simulink model "AppMain"  (R2021a)
settings: Solver=FixedStepDiscrete  StartTime=0.0  StopTime=0.02  FixedStep=10e-3  RelTol=1e-3
PreLoadFcn:
  | AppMain_data
values from neighbouring files (symbols this model uses):
  CtrlConst = struct    [AppMain_data.m]
  TaskTimeBase = struct    [AppMain_data.m]
undefined symbols (not defined in the file or in its folder): Lock, Open, Short
libraries: simulink x18, lib1 x6
(part 1 of 2)
settings Model: Creator=mdl4347  LastModifiedBy=13714
settings SolverCC: AlgebraicLoopSolver=TrustRegion
settings DataIOCC: ReturnWorkspaceOutputs=off
settings OptimizationCC: DefaultParameterBehavior=Inlined  InlineInvariantSignals=on  BufferReuse=off  GlobalBufferReuse=off  PassReuseOutputArgsAs=Individual arguments  OptimizeBlockOrder=speed  DifferentSizesBufferReuse=on  LabelGuidedReuse=on  EfficientTunableParamExpr=on
settings DebuggingCC: WriteAfterWriteMsg=EnableAllAsError  AlgebraicLoopMsg=error  IntegerOverflowMsg=error  ParameterUnderflowMsg=error  ParameterTunabilityLossMsg=error  BusObjectLabelMismatch=error  AllowSymbolicDim=off  ModelReferenceIOMsg=warning  PregeneratedLibrarySubsystemCodeDiagnostic=none  StrictBusMsg=ErrorOnBusTreatedAsVector  NonBusSignalsTreatedAsBus=error  SFInvalidInputDataAccessInChartInitDiag=error  SFTransitionOutsideNaturalParentDiag=error  SFUnreachableExecutionPathDiag=error  SFUndirectedBroadcastEventsDiag=error  SFTransitionActionBeforeConditionDiag=error  SFMachineParentedDataDiag=warning  IntegerSaturationMsg=error  ArithmeticOperatorsInVariantConditions=warning
settings HardwareCC: ProdBitPerPointer=32  ProdBitPerSizeT=32  ProdBitPerPtrDiffT=32  ProdLargestAtomicInteger=Long  ProdLargestAtomicFloat=Double  ProdWordSize=32  ProdHWDeviceType=ARM Compatible->ARM Cortex
settings ModelReferenceCC: ModelReferenceNumInstancesAllowed=Single
settings SFSimCC: SimUseLocalCustomCode=off  MATLABDynamicMemAlloc=off  CustomCodeUndefinedFunction=UseInterfaceOnly
settings RTWCC: SystemTargetFile=ert.tlc  GenCodeOnly=on  TemplateMakefile=ert_default_tmf  GenerateReport=on  RTWUseLocalCustomCode=off  RTWUseSimCustomCode=on  BuildConfiguration=Debug  IncludeHyperlinkInReport=on  PortableWordSizes=on  GenerateTraceInfo=on  GenerateTraceReport=on  GenerateTraceReportSl=on  GenerateTraceReportSf=on  GenerateTraceReportEml=on
settings CodeAppCC: ForceParamTrailComments=on  IgnoreCustomStorageClasses=off  SimulinkDataObjDesc=on  SFDataObjDesc=on  MATLABFcnDesc=on  MangleLength=4  CustomSymbolStrGlobalVar=$N$M  CustomSymbolStrType=$N$M_T  CustomSymbolStrFcn=$U$N$M$F  CustomSymbolStrMacro=$N$M  InsertBlockDesc=on  BlockCommentType=BlockSIDComment  StateflowObjectComments=on  EnableCustomComments=on  ReqsInCode=on
settings ERTTargetCC: TargetLangStandard=C99 (ISO)  GenerateSampleERTMain=on  IncludeMdlTerminateFcn=off  SuppressErrorStatus=on  SupportAbsoluteTime=off  PurelyIntegerCode=on  SupportNonFinite=off  SupportComplex=off  ERTCustomFileTemplate=example_file_process.tlc  GlobalDataDefinition=InSeparateSourceFile  GlobalDataReference=InSeparateHeaderFile  PreserveExpressionOrder=on  PreserveIfCondition=on  EnableSignedRightShifts=off  IndentStyle=Allman

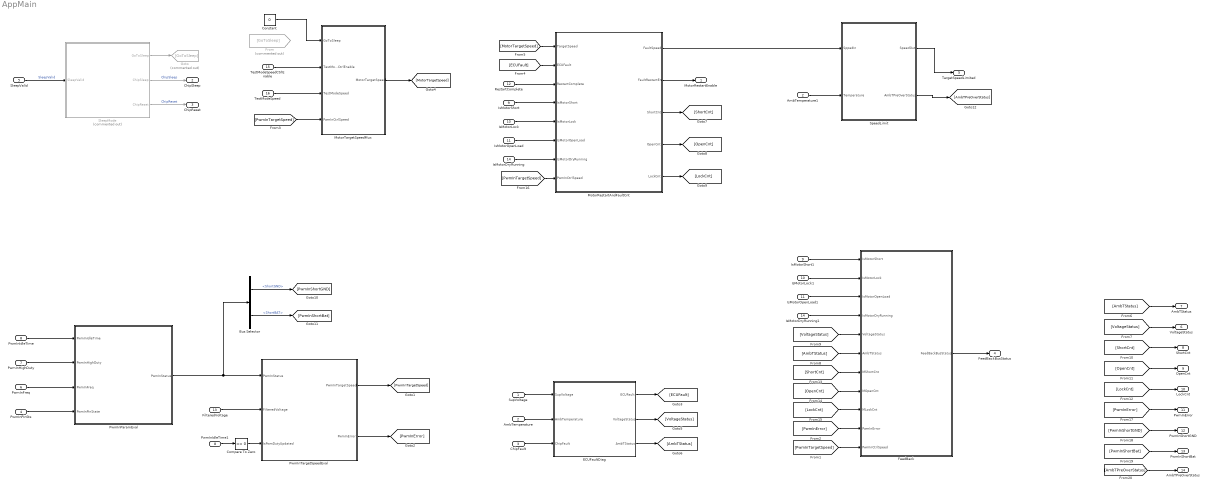
== system AppMain ==
  SupVoltage : Inport  OutDataTypeStr=int16
  AmbTemperature : Inport  Port=2  OutDataTypeStr=int16
  ChipFault : Inport  Port=3  OutDataTypeStr=boolean
  PwmInPinSts : Inport  Port=4  OutDataTypeStr=boolean
  SleepValid : Inport  Port=5  OutDataTypeStr=boolean
  PwmInFreq : Inport  Port=6  OutDataTypeStr=uint16
  PwmInHighDuty : Inport  Port=7  OutDataTypeStr=uint16
  PwmInIdleTime : Inport  Port=8  OutDataTypeStr=uint16
  IsMotorShort : Inport  Port=9  OutDataTypeStr=boolean
  IsMotorLock : Inport  Port=10  OutDataTypeStr=boolean
  IsMotorOpenLoad : Inport  Port=11  OutDataTypeStr=boolean
  RestartComplete : Inport  Port=12  OutDataTypeStr=boolean
  FilteredVoltage : Inport  Port=13  OutDataTypeStr=int16
  IsMotorDryRunning : Inport  Port=14  OutDataTypeStr=boolean
  TestModeSpeedCtrlEnable : Inport  Port=15  OutDataTypeStr=boolean
  TestModeSpeed : Inport  Port=16  OutDataTypeStr=int16
  AmbTemperature1 : InportShadow  Port=2  OutDataTypeStr=int16
  Bus Selector : BusSelector  OutputSignals=ShortGND,ShortBAT
  Compare To Zero : simulink/Logic and Bit Operations/Compare To Zero  relop===  OutDataTypeStr=boolean
  Constant : Constant  Value=0  OutDataTypeStr=boolean
  ECUFaultDiag : Subsystem  TreatAsAtomicUnit=on  SystemSampleTime=TaskTimeBase.FaultDiag
      settings: RTWFcnNameOpts=Use subsystem name  RTWFileNameOpts=Use subsystem name
  FeedBack : Subsystem  TreatAsAtomicUnit=on  SystemSampleTime=TaskTimeBase.FeedBack
      settings: RTWSystemCode=Nonreusable function  RTWFcnNameOpts=Use subsystem name  RTWFileNameOpts=Use subsystem name  FunctionInterfaceSpec=Allow arguments (Optimized)
  From : From  Commented=on  GotoTag=GoToSleep
  Goto : Goto  Commented=on  GotoTag=GoToSleep
  IsMotorDryRunning1 : InportShadow  Port=14  OutDataTypeStr=boolean
  IsMotorLock1 : InportShadow  Port=10  OutDataTypeStr=boolean
  IsMotorOpenLoad1 : InportShadow  Port=11  OutDataTypeStr=boolean
  IsMotorShort1 : InportShadow  Port=9  OutDataTypeStr=boolean
  MotorRestartAndFaultCnt : Subsystem  TreatAsAtomicUnit=on  SystemSampleTime=TaskTimeBase.SpeedCtrl
      settings: RTWFcnNameOpts=Use subsystem name  RTWFileNameOpts=Use subsystem name
  MotorTargetSpeedMux : Subsystem  TreatAsAtomicUnit=on  SystemSampleTime=TaskTimeBase.SpeedCtrl
      settings: RTWFcnNameOpts=Use subsystem name  RTWFileNameOpts=Use subsystem name
  PwmInIdleTime1 : InportShadow  Port=8  OutDataTypeStr=uint16
  PwmInParamEval : Subsystem  TreatAsAtomicUnit=on  SystemSampleTime=TaskTimeBase.PwmIn  RTWFcnName=PwmIn_5msTask
      settings: RTWSystemCode=Nonreusable function  RTWFcnNameOpts=Use subsystem name  RTWFileNameOpts=Use subsystem name
  PwmInTargetSpeedEval : Subsystem  TreatAsAtomicUnit=on  SystemSampleTime=TaskTimeBase.SpeedCtrl
      settings: RTWFcnNameOpts=Use subsystem name  RTWFileNameOpts=Use subsystem name
  SleepMode : Subsystem  Commented=on  TreatAsAtomicUnit=on  SystemSampleTime=TaskTimeBase.SleepMode
      settings: RTWFcnNameOpts=Use subsystem name  RTWFileNameOpts=Use subsystem name
  SpeedLimit : Subsystem  TreatAsAtomicUnit=on  SystemSampleTime=TaskTimeBase.SpeedCtrl
  MotorRestartEnable : Outport  OutDataTypeStr=boolean  VectorParamsAs1DForOutWhenUnconnected=off
  ChipSleep : Outport  Port=2  OutDataTypeStr=boolean  VectorParamsAs1DForOutWhenUnconnected=off
  ChipReset : Outport  Port=3  OutDataTypeStr=boolean  VectorParamsAs1DForOutWhenUnconnected=off
  FeedBackBusStatus : Outport  Port=4  OutDataTypeStr=boolean  VectorParamsAs1DForOutWhenUnconnected=off
  TargetSpeedLimited : Outport  Port=5  OutDataTypeStr=int16  VectorParamsAs1DForOutWhenUnconnected=off
  VoltageStatus : Outport  Port=6  VectorParamsAs1DForOutWhenUnconnected=off
  AmbTStatus : Outport  Port=7  VectorParamsAs1DForOutWhenUnconnected=off
  ShortCnt : Outport  Port=8  OutDataTypeStr=uint8  VectorParamsAs1DForOutWhenUnconnected=off
  OpenCnt : Outport  Port=9  OutDataTypeStr=uint8  VectorParamsAs1DForOutWhenUnconnected=off
  LockCnt : Outport  Port=10  OutDataTypeStr=uint8  VectorParamsAs1DForOutWhenUnconnected=off
  PwmInError : Outport  Port=11  OutDataTypeStr=boolean  VectorParamsAs1DForOutWhenUnconnected=off
  PwmInShortGND : Outport  Port=12  OutDataTypeStr=boolean  VectorParamsAs1DForOutWhenUnconnected=off
  PwmInShortBat : Outport  Port=13  OutDataTypeStr=boolean  VectorParamsAs1DForOutWhenUnconnected=off
  AmbTPreOverStatus : Outport  Port=14
  wires:
  SupVoltage/1 -> ECUFaultDiag/1(SupVoltage)
  ECUFaultDiag/1(ECUFault) -> [ECUFault]
  AmbTemperature/1 -> ECUFaultDiag/2(AmbTemperature)
  PwmInParamEval/1(PwmInStatus) -> Bus Selector/1, PwmInTargetSpeedEval/1(PwmInStatus)
  ChipFault/1 -> ECUFaultDiag/3(ChipFault)
  PwmInTargetSpeedEval/1(PwmInTargetSpeed) -> [PwmInTargetSpeed]
  PwmInIdleTime/1 -> PwmInParamEval/1(PwmInIdleTime)
  PwmInPinSts/1 -> PwmInParamEval/4(PwmInPinState)
  SleepValid/1 -> SleepMode/1(SleepValid)  "SleepValid"
  MotorRestartAndFaultCnt/2(FaultRestartEn) -> MotorRestartEnable/1
  SleepMode/2(ChipSleep) -> ChipSleep/1  "ChipSleep"
  SleepMode/3(ChipReset) -> ChipReset/1  "ChipReset"
  PwmInFreq/1 -> PwmInParamEval/3(PwmInFreq)
  PwmInHighDuty/1 -> PwmInParamEval/2(PwmInHighDuty)
  IsMotorShort/1 -> MotorRestartAndFaultCnt/4(IsMotorShort)
  IsMotorOpenLoad/1 -> MotorRestartAndFaultCnt/6(IsMotorOpenLoad)
  IsMotorLock/1 -> MotorRestartAndFaultCnt/5(IsMotorLock)
  RestartComplete/1 -> MotorRestartAndFaultCnt/3(RestartComplete)
  ECUFaultDiag/2(VoltageStatus) -> [VoltageStatus]
  ECUFaultDiag/3(AmbTStatus) -> [AmbTStatus]
  FeedBack/1(FeedBackBusStatus) -> FeedBackBusStatus/1
  MotorRestartAndFaultCnt/1(FaultSpeed) -> SpeedLimit/1(SppedIn)
  AmbTemperature1/1 -> SpeedLimit/2(Temperature)
  SpeedLimit/1(SpeedOut) -> TargetSpeedLimited/1
  FilteredVoltage/1 -> PwmInTargetSpeedEval/2(FilteredVoltage)
  Compare To Zero/1 -> PwmInTargetSpeedEval/3(IsPwmDutyUpdated)
  IsMotorDryRunning/1 -> MotorRestartAndFaultCnt/7(IsMotorDryRunning)
  MotorRestartAndFaultCnt/4(OpenCnt) -> [OpenCnt]
  MotorRestartAndFaultCnt/5(LockCnt) -> [LockCnt]
  PwmInTargetSpeedEval/2(PwmInError) -> [PwmInError]
  MotorRestartAndFaultCnt/3(ShortCnt) -> [ShortCnt]
  SleepMode/1(GoToSleep) -> Goto/1
  PwmInIdleTime1/1 -> Compare To Zero/1
  [PwmInTargetSpeed] -> FeedBack/11(PwmInCtrlSpeed)
  [PwmInError] -> FeedBack/10(PwmInError)
  [PwmInTargetSpeed] -> MotorTargetSpeedMux/4(PwmInCtrlSpeed)
  TestModeSpeedCtrlEnable/1 -> MotorTargetSpeedMux/2(TestModeSpeedCtrlEnable)
  TestModeSpeed/1 -> MotorTargetSpeedMux/3(TestModeSpeed)
  [ECUFault] -> MotorRestartAndFaultCnt/2(ECUFault)
  MotorTargetSpeedMux/1(MotorTargetSpeed) -> [MotorTargetSpeed]
  [MotorTargetSpeed] -> MotorRestartAndFaultCnt/1(TargetSpeed)
  [AmbTStatus] -> AmbTStatus/1
  [VoltageStatus] -> VoltageStatus/1
  [AmbTStatus] -> FeedBack/6(AmbTStatus)
  [VoltageStatus] -> FeedBack/5(VoltageStatus)
  IsMotorShort1/1 -> FeedBack/1(IsMotorShort)
  IsMotorLock1/1 -> FeedBack/2(IsMotorLock)
  IsMotorOpenLoad1/1 -> FeedBack/3(IsMotorOpenLoad)
  IsMotorDryRunning1/1 -> FeedBack/4(IsMotorDryRunning)
  [ShortCnt] -> ShortCnt/1
  [OpenCnt] -> OpenCnt/1
  [LockCnt] -> LockCnt/1
  [ShortCnt] -> FeedBack/7(MShortCnt)
  [OpenCnt] -> FeedBack/8(MOpenCnt)
  [LockCnt] -> FeedBack/9(MLockCnt)
  [PwmInTargetSpeed] -> MotorRestartAndFaultCnt/8(PwmInCtrlSpeed)
  Bus Selector/1 -> [PwmInShortGND]  "<ShortGND>"
  Bus Selector/2 -> [PwmInShortBat]  "<ShortBAT>"
  [PwmInError] -> PwmInError/1
  [PwmInShortGND] -> PwmInShortGND/1
  [PwmInShortBat] -> PwmInShortBat/1
  Constant/1 -> MotorTargetSpeedMux/1(GoToSleep)
  SpeedLimit/2(AmbTPreOverStatus) -> [AmbTPreOverStatus]
  [AmbTPreOverStatus] -> AmbTPreOverStatus/1

== system AppMain/ECUFaultDiag ==
  SupVoltage : Inport  OutDataTypeStr=int16
  AmbTemperature : Inport  Port=2
  ChipFault : Inport  Port=3
  AmbTemperatureDiag : Subsystem  TreatAsAtomicUnit=on
      settings: RTWFcnNameOpts=Use subsystem name
  Compare To Constant : simulink/Logic and Bit Operations/Compare To Constant  relop=~=  const=0  OutDataTypeStr=boolean
  Compare To Constant1 : simulink/Logic and Bit Operations/Compare To Constant  relop=~=  const=0  OutDataTypeStr=boolean
  Logical Operator : Logic  Operator=OR  Inputs=3  AllPortsSameDT=off  OutDataTypeStr=boolean
  VoltageDiag : Subsystem  TreatAsAtomicUnit=on
      settings: RTWFcnNameOpts=Use subsystem name
  ECUFault : Outport  VectorParamsAs1DForOutWhenUnconnected=off
  VoltageStatus : Outport  Port=2  OutDataTypeStr=int8  VectorParamsAs1DForOutWhenUnconnected=off
  AmbTStatus : Outport  Port=3  OutDataTypeStr=int8  VectorParamsAs1DForOutWhenUnconnected=off
  wires:
  SupVoltage/1 -> VoltageDiag/1(Voltage)
  AmbTemperature/1 -> AmbTemperatureDiag/1(AmbTemperature)
  AmbTemperatureDiag/1(AmbTStatus) -> Compare To Constant1/1, AmbTStatus/1  "AmbTStatus"
  VoltageDiag/1(VoltageStatus) -> VoltageStatus/1, Compare To Constant/1  "VoltageStatus"
  ChipFault/1 -> Logical Operator/3  "ChipFualt"
  Compare To Constant/1 -> Logical Operator/1
  Compare To Constant1/1 -> Logical Operator/2
  Logical Operator/1 -> ECUFault/1  "ECUFault"

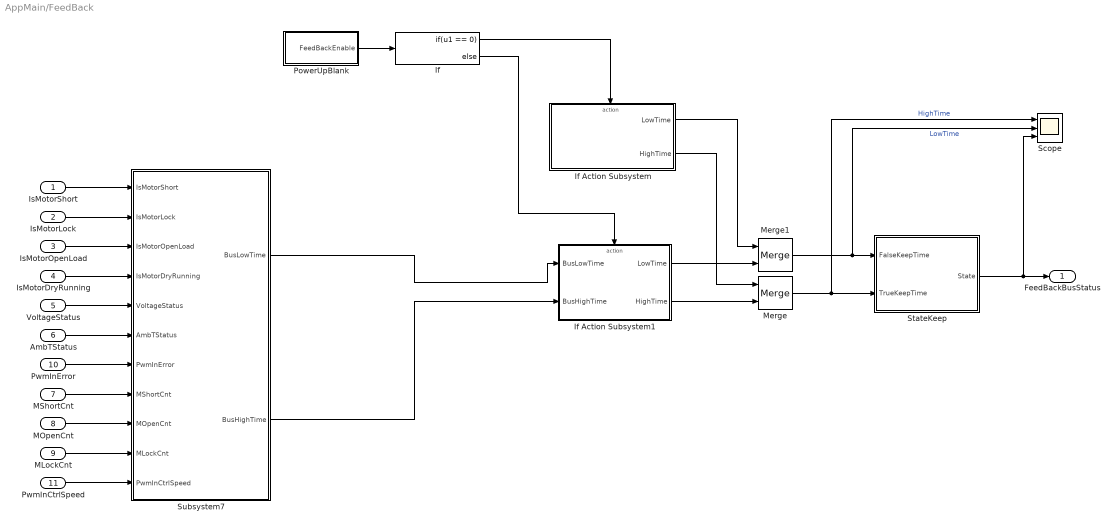
== system AppMain/FeedBack ==
  IsMotorShort : Inport  OutDataTypeStr=boolean
  IsMotorLock : Inport  Port=2  OutDataTypeStr=boolean
  IsMotorOpenLoad : Inport  Port=3  OutDataTypeStr=boolean
  IsMotorDryRunning : Inport  Port=4  OutDataTypeStr=boolean
  VoltageStatus : Inport  Port=5  OutDataTypeStr=int8
  AmbTStatus : Inport  Port=6  OutDataTypeStr=int8
  MShortCnt : Inport  Port=7  OutDataTypeStr=uint8
  MOpenCnt : Inport  Port=8  OutDataTypeStr=uint8
  MLockCnt : Inport  Port=9  OutDataTypeStr=uint8
  PwmInError : Inport  Port=10  OutDataTypeStr=boolean
  PwmInCtrlSpeed : Inport  Port=11  OutDataTypeStr=int16
  If : If  IfExpression=u1 == 0
  If Action Subsystem : Subsystem  TreatAsAtomicUnit=on
  If Action Subsystem1 : Subsystem  TreatAsAtomicUnit=on
  Merge : Merge
  Merge1 : Merge
  PowerUpBlank : Subsystem
  Scope : Scope  NumInputPorts=3
  StateKeep : Stateflow chart  TreatAsAtomicUnit=on
  Subsystem7 : Subsystem
  FeedBackBusStatus : Outport  OutDataTypeStr=boolean  VectorParamsAs1DForOutWhenUnconnected=off
  wires:
  StateKeep/1(State) -> FeedBackBusStatus/1, Scope/3
  IsMotorShort/1 -> Subsystem7/1(IsMotorShort)
  IsMotorLock/1 -> Subsystem7/2(IsMotorLock)
  IsMotorOpenLoad/1 -> Subsystem7/3(IsMotorOpenLoad)
  IsMotorDryRunning/1 -> Subsystem7/4(IsMotorDryRunning)
  VoltageStatus/1 -> Subsystem7/5(VoltageStatus)
  AmbTStatus/1 -> Subsystem7/6(AmbTStatus)
  PwmInError/1 -> Subsystem7/7(PwmInError)
  PowerUpBlank/1(FeedBackEnable) -> If/1
  If/1 -> If Action Subsystem/Action
  If/2 -> If Action Subsystem1/Action
  Subsystem7/1(BusLowTime) -> If Action Subsystem1/1(BusLowTime)
  Subsystem7/2(BusHighTime) -> If Action Subsystem1/2(BusHighTime)
  If Action Subsystem1/2(HighTime) -> Merge/2
  If Action Subsystem/2(HighTime) -> Merge/1
  If Action Subsystem1/1(LowTime) -> Merge1/2
  If Action Subsystem/1(LowTime) -> Merge1/1
  Merge1/1 -> StateKeep/1(FalseKeepTime), Scope/2  "LowTime"
  Merge/1 -> StateKeep/2(TrueKeepTime), Scope/1  "HighTime"
  MShortCnt/1 -> Subsystem7/8(MShortCnt)
  MOpenCnt/1 -> Subsystem7/9(MOpenCnt)
  MLockCnt/1 -> Subsystem7/10(MLockCnt)
  PwmInCtrlSpeed/1 -> Subsystem7/11(PwmInCtrlSpeed)

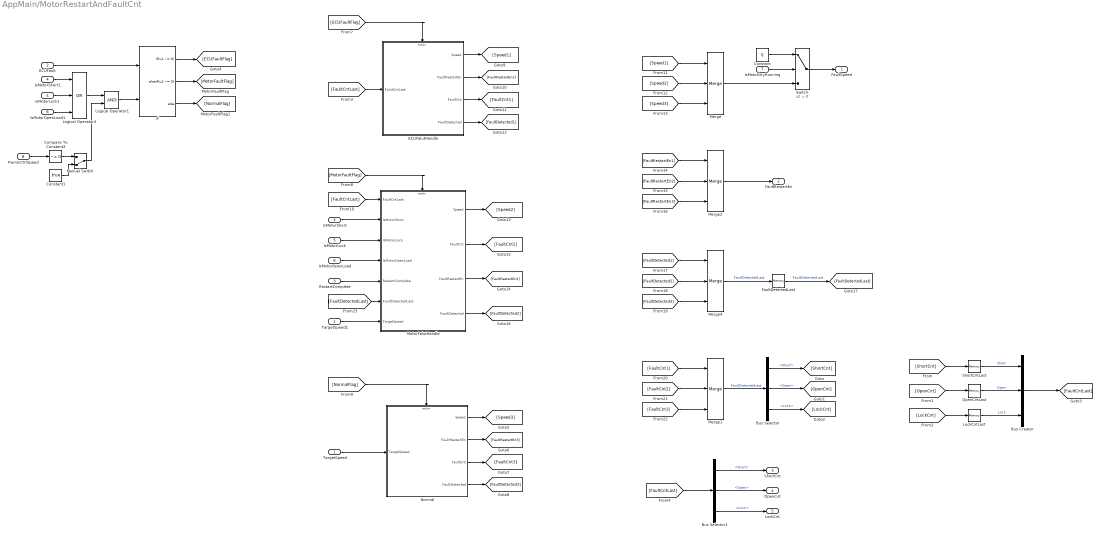
== system AppMain/MotorRestartAndFaultCnt ==
  TargetSpeed : Inport  OutDataTypeStr=int16
  ECUFault : Inport  Port=2
  RestartComplete : Inport  Port=3  OutDataTypeStr=boolean
  IsMotorShort : Inport  Port=4  OutDataTypeStr=boolean
  IsMotorLock : Inport  Port=5  OutDataTypeStr=boolean
  IsMotorOpenLoad : Inport  Port=6  OutDataTypeStr=boolean
  IsMotorDryRunning : Inport  Port=7  OutDataTypeStr=boolean
  PwmInCtrlSpeed : Inport  Port=8  OutDataTypeStr=int16
  Bus Creator : BusCreator  Inputs=3  OutDataTypeStr=Bus: MotorFaultCnt_t  NonVirtualBus=on
      settings: InheritFromInputs=off
  Bus Selector : BusSelector  OutputSignals=Short,Open,Lock
  Bus Selector1 : BusSelector  OutputSignals=Short,Open,Lock
  Compare To Constant3 : simulink/Logic and Bit Operations/Compare To Constant  relop=~=  const=0  OutDataTypeStr=boolean
  Constant : Constant  Value=0  OutDataTypeStr=int16
  Constant1 : Constant  Value=true
  ECUFalutHandle : Subsystem  TreatAsAtomicUnit=on
  FaultDetectedLast : Memory  InitialCondition=1  InheritSampleTime=on
  If : If  NumInputs=2  IfExpression=u1 ~= 0  ElseIfExpressions=u2 ~= 0
  IsMotorLock1 : InportShadow  Port=5  OutDataTypeStr=boolean
  IsMotorOpenLoad1 : InportShadow  Port=6  OutDataTypeStr=boolean
  IsMotorShort1 : InportShadow  Port=4  OutDataTypeStr=boolean
  LockCntLast : Memory  InheritSampleTime=on
  Logical Operator1 : Logic  AllPortsSameDT=off  OutDataTypeStr=boolean
  Logical Operator4 : Logic  Operator=OR  Inputs=3  AllPortsSameDT=off  OutDataTypeStr=boolean
  Manual Switch : ManualSwitch  CurrentSetting=0
  Merge{,1..2,4} (4 alike) : Merge  Inputs=3
  MotorFalutHandle : Subsystem  TreatAsAtomicUnit=on
  Normal : Subsystem  TreatAsAtomicUnit=on
  OpenCntLast : Memory  InheritSampleTime=on
  ShortCntLast : Memory  InheritSampleTime=on
  Switch : Switch  Criteria=u2 > Threshold
  TargetSpeed1 : InportShadow  OutDataTypeStr=int16
  FaultSpeed : Outport  OutDataTypeStr=int16  VectorParamsAs1DForOutWhenUnconnected=off
  FaultRestartEn : Outport  Port=2  OutDataTypeStr=boolean  VectorParamsAs1DForOutWhenUnconnected=off
  ShortCnt : Outport  Port=3  OutDataTypeStr=uint8  VectorParamsAs1DForOutWhenUnconnected=off
  OpenCnt : Outport  Port=4  OutDataTypeStr=uint8  VectorParamsAs1DForOutWhenUnconnected=off
  LockCnt : Outport  Port=5  OutDataTypeStr=uint8  VectorParamsAs1DForOutWhenUnconnected=off
  wires:
  ECUFault/1 -> If/1
  IsMotorShort/1 -> MotorFalutHandle/2(IsMotorShort)
  IsMotorLock/1 -> MotorFalutHandle/3(IsMotorLock)
  IsMotorOpenLoad/1 -> MotorFalutHandle/4(IsMotorOpenLoad)
  Merge/1 -> Switch/3
  Merge2/1 -> FaultRestartEn/1
  RestartComplete/1 -> MotorFalutHandle/5(RestartComplete)
  [FaultCntLast] -> ECUFalutHandle/1(FalutCntLast)
  TargetSpeed/1 -> Normal/1(TargetSpeed)
  Merge4/1 -> FaultDetectedLast/1  "FaultDetectedLast"
  LockCntLast/1 -> Bus Creator/3  "Lock"
  OpenCntLast/1 -> Bus Creator/2  "Open"
  ShortCntLast/1 -> Bus Creator/1  "Short"
  Bus Selector/2 -> [OpenCnt]  "<Open>"
  Bus Selector/1 -> [ShortCnt]  "<Short>"
  Bus Selector/3 -> [LockCnt]  "<Lock>"
  IsMotorDryRunning/1 -> Switch/2
  Constant/1 -> Switch/1
  Switch/1 -> FaultSpeed/1
  PwmInCtrlSpeed/1 -> Compare To Constant3/1
  [ShortCnt] -> ShortCntLast/1
  [OpenCnt] -> OpenCntLast/1
  [LockCnt] -> LockCntLast/1
  IsMotorShort1/1 -> Logical Operator4/1
  IsMotorLock1/1 -> Logical Operator4/2
  IsMotorOpenLoad1/1 -> Logical Operator4/3
  If/1 -> [ECUFaultFlag]
  If/2 -> [MotorFaultFlag]
  If/3 -> [NormalFlag]
  [ECUFaultFlag] -> ECUFalutHandle/Action
  [MotorFaultFlag] -> MotorFalutHandle/Action
  [NormalFlag] -> Normal/Action
  TargetSpeed1/1 -> MotorFalutHandle/7(TargetSpeed)
  Normal/1(Speed) -> [Speed3]
  Normal/2(FaultRestartEn) -> [FaultRestartEn3]
  Normal/4(FaultDetected) -> [FaultDetected3]
  [FaultCntLast] -> MotorFalutHandle/1(FaultCntLast)
  ECUFalutHandle/1(Speed) -> [Speed1]
  ECUFalutHandle/2(FaultRestartEn) -> [FaultRestartEn1]
  ECUFalutHandle/3(FaultCnt) -> [FaultCnt1]
  ECUFalutHandle/4(FaultDetected) -> [FaultDetected1]
  MotorFalutHandle/1(Speed) -> [Speed2]
  MotorFalutHandle/4(FaultDetected) -> [FaultDetected2]
  [Speed1] -> Merge/1
  [Speed2] -> Merge/2
  [Speed3] -> Merge/3
  [FaultRestartEn3] -> Merge2/3
  [FaultRestartEn2] -> Merge2/2
  [FaultRestartEn1] -> Merge2/1
  [FaultDetected2] -> Merge4/2
  [FaultDetected1] -> Merge4/1
  [FaultDetected3] -> Merge4/3
  FaultDetectedLast/1 -> [FaultDetectedLast]  "FaultDetectedLast"
  [FaultCnt1] -> Merge1/1
  [FaultCnt2] -> Merge1/2
  [FaultCnt3] -> Merge1/3
  Merge1/1 -> Bus Selector/1  "FaultDetectedLast"
  [FaultDetectedLast] -> MotorFalutHandle/6(FaultDetectedLast)
  Bus Creator/1 -> [FaultCntLast]
  MotorFalutHandle/3(FaultRestartEn) -> [FaultRestartEn2]
  MotorFalutHandle/2(FaultCnt) -> [FaultCnt2]
  Normal/3(FaultCnt) -> [FaultCnt3]
  Bus Selector1/1 -> ShortCnt/1  "<Short>"
  Bus Selector1/2 -> OpenCnt/1  "<Open>"
  Bus Selector1/3 -> LockCnt/1  "<Lock>"
  [FaultCntLast] -> Bus Selector1/1
  Logical Operator4/1 -> Logical Operator1/1
  Compare To Constant3/1 -> Manual Switch/1
  Constant1/1 -> Manual Switch/2
  Logical Operator1/1 -> If/2
  Manual Switch/1 -> Logical Operator1/2

== system AppMain/MotorTargetSpeedMux ==
  GoToSleep : Inport  OutDataTypeStr=boolean
  TestModeSpeedCtrlEnable : Inport  Port=2  OutDataTypeStr=boolean
  TestModeSpeed : Inport  Port=3  OutDataTypeStr=int16
  PwmInCtrlSpeed : Inport  Port=4  OutDataTypeStr=int16
  Constant : Constant  Value=0  OutDataTypeStr=int16
  Switch1 : Switch  Criteria=u2 ~= 0
  Switch2 : Switch  Criteria=u2 ~= 0
  MotorTargetSpeed : Outport  OutDataTypeStr=int16  VectorParamsAs1DForOutWhenUnconnected=off
  wires:
  TestModeSpeedCtrlEnable/1 -> Switch1/2
  TestModeSpeed/1 -> Switch1/1
  PwmInCtrlSpeed/1 -> Switch1/3
  Switch1/1 -> Switch2/3
  GoToSleep/1 -> Switch2/2
  Constant/1 -> Switch2/1
  Switch2/1 -> MotorTargetSpeed/1  "MotorTargetSpeed"

== system AppMain/PwmInParamEval ==
  PwmInIdleTime : Inport  OutDataTypeStr=uint16
  PwmInHighDuty : Inport  Port=2  OutDataTypeStr=uint16
  PwmInFreq : Inport  Port=3  OutDataTypeStr=uint16
  PwmInPinState : Inport  Port=4  OutDataTypeStr=boolean
  Bus Creator : BusCreator  Inputs=4  OutDataTypeStr=Bus: PwmInStatus_t
  PwmInshortDetect : Subsystem  TreatAsAtomicUnit=on
      settings: RTWSystemCode=Nonreusable function  RTWFcnNameOpts=Use subsystem name
  PwmInStatus : Outport  VectorParamsAs1DForOutWhenUnconnected=off
  wires:
  PwmInshortDetect/1(shortGND) -> Bus Creator/1  "ShortGND"
  PwmInshortDetect/2(shortBat) -> Bus Creator/2  "ShortBAT"
  PwmInHighDuty/1 -> Bus Creator/4  "HighDuty"
  PwmInFreq/1 -> Bus Creator/3  "Freq"
  PwmInIdleTime/1 -> PwmInshortDetect/1(PwmInIdleTime)  "PwmInIdleTime"
  PwmInPinState/1 -> PwmInshortDetect/2(PwmInPinState)  "PwmInPinState"
  Bus Creator/1 -> PwmInStatus/1

== system AppMain/PwmInTargetSpeedEval ==
  PwmInStatus : Inport
  FilteredVoltage : Inport  Port=2  OutDataTypeStr=int16
  IsPwmDutyUpdated : Inport  Port=3  OutDataTypeStr=boolean
  If : If  IfExpression=u1 ~= 0
  Merge : Merge
  Merge1 : Merge
  Merge2 : Merge
  NormalState : Subsystem  TreatAsAtomicUnit=on
  PowerOnBlankState : Subsystem  TreatAsAtomicUnit=on
  PowerOnBlankTimeCnt : Memory  InheritSampleTime=on
  PowerOnBlankTimeThreshold : Constant  Value=CtrlConst.SpeedCtrl.PwmIn.PowerOnBlankTime  OutDataTypeStr=uint16
  Relational Operator : RelationalOperator  Operator=<  OutDataTypeStr=boolean  RndMeth=Simplest
  PwmInTargetSpeed : Outport  OutDataTypeStr=int16  VectorParamsAs1DForOutWhenUnconnected=off
  PwmInError : Outport  Port=2  OutDataTypeStr=boolean  VectorParamsAs1DForOutWhenUnconnected=off
  wires:
  PowerOnBlankTimeThreshold/1 -> Relational Operator/2
  PowerOnBlankTimeCnt/1 -> NormalState/1(PowerOnCntIn), PowerOnBlankState/1(PowerOnCntIn), Relational Operator/1  "PowerOnCntLast"
  Relational Operator/1 -> If/1  "InPowerOnState"
  If/1 -> PowerOnBlankState/Action
  If/2 -> NormalState/Action
  PwmInStatus/1 -> NormalState/2(PwmInStatus)  "PwmInStatus"
  Merge/1 -> PowerOnBlankTimeCnt/1
  PowerOnBlankState/1(PowerOnCntOut) -> Merge/1
  NormalState/1(PowerOnCntOut) -> Merge/2
  Merge1/1 -> PwmInTargetSpeed/1  "PwmInTargetSpeed"
  PowerOnBlankState/2(TargetSpeed) -> Merge1/1
  NormalState/2(TargetSpeed) -> Merge1/2
  PowerOnBlankState/3(PwmInError) -> Merge2/1
  Merge2/1 -> PwmInError/1  "PwmInError"
  NormalState/3(PwmInError) -> Merge2/2
  FilteredVoltage/1 -> NormalState/3(FilteredVoltage)
  IsPwmDutyUpdated/1 -> NormalState/4(IsPwmDutyUpdated)  "IsPwmDutyUpdated"

== system AppMain/SleepMode ==
  SleepValid : Inport  OutDataTypeStr=boolean
  SleepMode : Stateflow chart  TreatAsAtomicUnit=on
  SleepModeValidCntTHR : Constant  Value=CtrlConst.SpeedMode.ValidCntTHR
  SleepModeWaitTimeTHR : Constant  Value=CtrlConst.SpeedMode.WaitTimeTHR
  GoToSleep : Outport  OutDataTypeStr=boolean  VectorParamsAs1DForOutWhenUnconnected=off
  ChipSleep : Outport  Port=2  OutDataTypeStr=boolean  VectorParamsAs1DForOutWhenUnconnected=off
  ChipReset : Outport  Port=3  OutDataTypeStr=boolean  VectorParamsAs1DForOutWhenUnconnected=off
  wires:
  SleepValid/1 -> SleepMode/1(SleepValid)  "SleepValid"
  SleepMode/1(GoToSleep) -> GoToSleep/1  "GoToSleep"
  SleepMode/2(ChipSleep) -> ChipSleep/1  "ChipSleep"
  SleepMode/3(ChipReset) -> ChipReset/1  "ChipReset"
  SleepModeValidCntTHR/1 -> SleepMode/2(SleepValidCntTHR)
  SleepModeWaitTimeTHR/1 -> SleepMode/3(SleepWaitTimeTHR)

== system AppMain/SpeedLimit ==
  SppedIn : Inport  OutDataTypeStr=int16
  Temperature : Inport  Port=2  OutDataTypeStr=int16
  AmbTPreOverDiag : lib1/TemperaturSstate  LowEntryTHR=CtrlConst.FaultDiag.AmbTemperature.THR.LowEntry  LowExitTHR=CtrlConst.FaultDiag.AmbTemperature.THR.LowExit  HighEntryTHR=CtrlConst.FaultDiag.AmbTemperature.THR.PreOverEntry  HighExitTHR=CtrlConst.FaultDiag.AmbTemperature.THR.PreOverExit  DelayCntTHR=CtrlConst.FaultDiag.AmbTemperature.PreOverFilterTime  LongDelayCntTHR=CtrlConst.FaultDiag.AmbTemperature.LongFilterTime
      settings: SourceProductName=lib1
  AmbTPreOverMaxSpeed : Constant  Value=CtrlConst.SpeedCtrl.PwmIn.TargetSpeed.Max*6/10  OutDataTypeStr=int16
  Relational Operator : RelationalOperator  Operator=<  OutDataTypeStr=boolean  RndMeth=Simplest
  Switch : Switch  Criteria=u2 > Threshold
  Switch1 : Switch  Criteria=u2 > Threshold
  SpeedOut : Outport  OutDataTypeStr=int16  VectorParamsAs1DForOutWhenUnconnected=off
  AmbTPreOverStatus : Outport  Port=2
  wires:
  Temperature/1 -> AmbTPreOverDiag/1
  SppedIn/1 -> Switch1/3, Relational Operator/2, Switch/3
  Switch/1 -> SpeedOut/1
  AmbTPreOverDiag/1 -> AmbTPreOverStatus/1, Switch/2  "AmbTStatus"
  AmbTPreOverMaxSpeed/1 -> Switch1/1, Relational Operator/1
  Relational Operator/1 -> Switch1/2
  Switch1/1 -> Switch/1

== system AppMain/ECUFaultDiag/AmbTemperatureDiag ==
  AmbTemperature : Inport
  TemperaturState : lib1/TemperaturSstate  LowEntryTHR=CtrlConst.FaultDiag.AmbTemperature.THR.LowEntry  LowExitTHR=CtrlConst.FaultDiag.AmbTemperature.THR.LowExit  HighEntryTHR=CtrlConst.FaultDiag.AmbTemperature.THR.OverEntry  HighExitTHR=CtrlConst.FaultDiag.AmbTemperature.THR.OverExit  DelayCntTHR=CtrlConst.FaultDiag.AmbTemperature.FilterTime  LongDelayCntTHR=CtrlConst.FaultDiag.AmbTemperature.LongFilterTime
      settings: SourceProductName=lib1
  AmbTStatus : Outport  VectorParamsAs1DForOutWhenUnconnected=off
  wires:
  AmbTemperature/1 -> TemperaturState/1
  TemperaturState/1 -> AmbTStatus/1  "AmbTStatus"

== system AppMain/ECUFaultDiag/VoltageDiag ==
  Voltage : Inport
  VoltageDiag : lib1/HysteresisState  LowEntryTHR=CtrlConst.FaultDiag.Voltage.THR.LowEntry  LowExitTHR=CtrlConst.FaultDiag.Voltage.THR.LowExit  HighEntryTHR=CtrlConst.FaultDiag.Voltage.THR.HighEntry  HighExitTHR=CtrlConst.FaultDiag.Voltage.THR.HighExit  DelayCntTHR=CtrlConst.FaultDiag.Voltage.FilterTime
      settings: SourceProductName=lib1
  VoltageStatus : Outport  VectorParamsAs1DForOutWhenUnconnected=off
  wires:
  Voltage/1 -> VoltageDiag/1
  VoltageDiag/1 -> VoltageStatus/1  "VoltageStatus"

== system AppMain/FeedBack/If Action Subsystem ==
  Action Port : ActionPort  ActionPortLabel=if(u1 == 0)
  Constant : Constant  Value=0  OutDataTypeStr=uint16
  Constant1 : Constant  OutDataTypeStr=uint16
  LowTime : Outport  VectorParamsAs1DForOutWhenUnconnected=off
  HighTime : Outport  Port=2  VectorParamsAs1DForOutWhenUnconnected=off
  wires:
  Constant/1 -> LowTime/1
  Constant1/1 -> HighTime/1

== system AppMain/FeedBack/If Action Subsystem1 ==
  BusLowTime : Inport
  BusHighTime : Inport  Port=2
  Action Port : ActionPort  ActionPortLabel=else
  LowTime : Outport  VectorParamsAs1DForOutWhenUnconnected=off
  HighTime : Outport  Port=2  VectorParamsAs1DForOutWhenUnconnected=off
  wires:
  BusLowTime/1 -> LowTime/1
  BusHighTime/1 -> HighTime/1

== system AppMain/FeedBack/PowerUpBlank ==
  Constant : Constant  OutDataTypeStr=boolean
  Constant1 : Constant  Value=CtrlConst.FeedBack.PowerUpBlankTime  OutDataTypeStr=uint16
  Constant2 : Constant  Value=0  OutDataTypeStr=uint16
  Display : Display
  PowerUpBlank : lib1/FeedBackDelay  SystemSampleTime=-1  VariantActivationTime=update diagram  Latency=0  AutoFrameSizeCalculation=off
      settings: SourceProductName=lib1
  FeedBackEnable : Outport  VectorParamsAs1DForOutWhenUnconnected=off
  wires:
  Constant1/1 -> PowerUpBlank/1
  PowerUpBlank/1 -> FeedBackEnable/1, Display/1  "FeedBackEnable"
  Constant/1 -> PowerUpBlank/2
  Constant2/1 -> PowerUpBlank/3

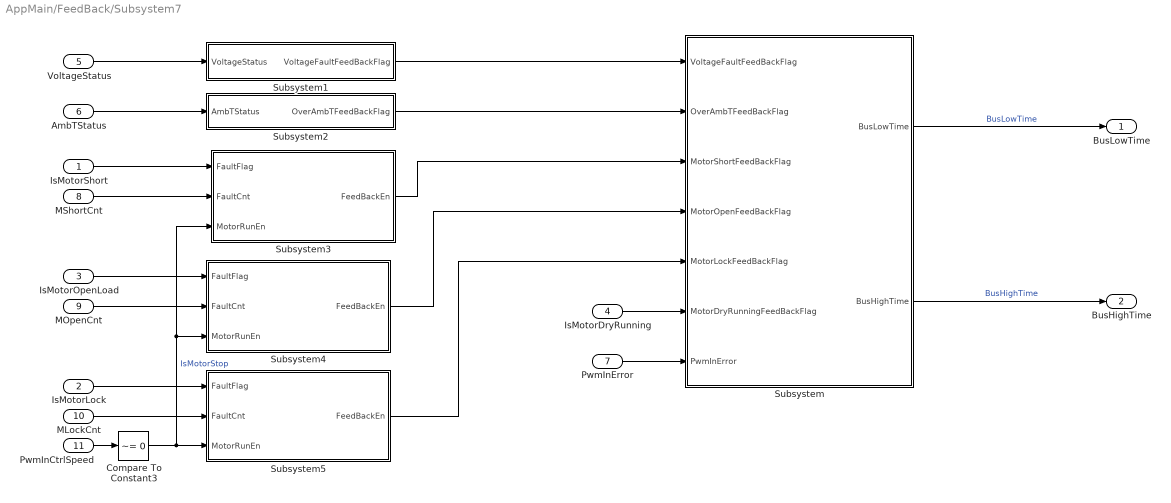
== system AppMain/FeedBack/Subsystem7 ==
  IsMotorShort : Inport  OutDataTypeStr=boolean
  IsMotorLock : Inport  Port=2  OutDataTypeStr=boolean
  IsMotorOpenLoad : Inport  Port=3  OutDataTypeStr=boolean
  IsMotorDryRunning : Inport  Port=4  OutDataTypeStr=boolean
  VoltageStatus : Inport  Port=5  OutDataTypeStr=int8
  AmbTStatus : Inport  Port=6  OutDataTypeStr=int8
  PwmInError : Inport  Port=7  OutDataTypeStr=boolean
  MShortCnt : Inport  Port=8  OutDataTypeStr=uint8
  MOpenCnt : Inport  Port=9  OutDataTypeStr=uint8
  MLockCnt : Inport  Port=10  OutDataTypeStr=uint8
  PwmInCtrlSpeed : Inport  Port=11  OutDataTypeStr=int16
  Compare To Constant3 : simulink/Logic and Bit Operations/Compare To Constant  relop=~=  const=0  OutDataTypeStr=boolean
  Subsystem : Subsystem
  Subsystem1 : Subsystem
  Subsystem2 : Subsystem
  Subsystem3 : Subsystem
  Subsystem4 : Subsystem
  Subsystem5 : Subsystem
  BusLowTime : Outport  VectorParamsAs1DForOutWhenUnconnected=off
  BusHighTime : Outport  Port=2  VectorParamsAs1DForOutWhenUnconnected=off
  wires:
  Subsystem1/1(VoltageFaultFeedBackFlag) -> Subsystem/1(VoltageFaultFeedBackFlag)
  VoltageStatus/1 -> Subsystem1/1(VoltageStatus)
  IsMotorDryRunning/1 -> Subsystem/6(MotorDryRunningFeedBackFlag)
  Subsystem2/1(OverAmbTFeedBackFlag) -> Subsystem/2(OverAmbTFeedBackFlag)
  Subsystem/1(BusLowTime) -> BusLowTime/1  "BusLowTime"
  Subsystem/2(BusHighTime) -> BusHighTime/1  "BusHighTime"
  AmbTStatus/1 -> Subsystem2/1(AmbTStatus)
  PwmInError/1 -> Subsystem/7(PwmInError)
  Subsystem4/1(FeedBackEn) -> Subsystem/4(MotorOpenFeedBackFlag)
  Subsystem5/1(FeedBackEn) -> Subsystem/5(MotorLockFeedBackFlag)
  PwmInCtrlSpeed/1 -> Compare To Constant3/1
  Compare To Constant3/1 -> Subsystem4/3(MotorRunEn), Subsystem3/3(MotorRunEn), Subsystem5/3(MotorRunEn)  "IsMotorStop"
  IsMotorShort/1 -> Subsystem3/1(FaultFlag)
  MShortCnt/1 -> Subsystem3/2(FaultCnt)
  Subsystem3/1(FeedBackEn) -> Subsystem/3(MotorShortFeedBackFlag)
  IsMotorOpenLoad/1 -> Subsystem4/1(FaultFlag)
  MOpenCnt/1 -> Subsystem4/2(FaultCnt)
  IsMotorLock/1 -> Subsystem5/1(FaultFlag)
  MLockCnt/1 -> Subsystem5/2(FaultCnt)

== system AppMain/MotorRestartAndFaultCnt/ECUFalutHandle ==
  FalutCntLast : Inport  OutDataTypeStr=Bus: MotorFaultCnt_t
  Action Port : ActionPort  ActionPortLabel=if(u1 ~= 0)
  Constant : Constant  Value=0  OutDataTypeStr=int16
  Constant1 : Constant  OutDataTypeStr=boolean
  Constant2 : Constant  Value=0  OutDataTypeStr=boolean
  Speed : Outport  OutDataTypeStr=int16  VectorParamsAs1DForOutWhenUnconnected=off
  FaultRestartEn : Outport  Port=2  OutDataTypeStr=boolean  VectorParamsAs1DForOutWhenUnconnected=off
  FaultCnt : Outport  Port=3  OutDataTypeStr=Bus: MotorFaultCnt_t  VectorParamsAs1DForOutWhenUnconnected=off
  FaultDetected : Outport  Port=4  OutDataTypeStr=boolean  VectorParamsAs1DForOutWhenUnconnected=off
  wires:
  Constant/1 -> Speed/1
  Constant2/1 -> FaultRestartEn/1
  FalutCntLast/1 -> FaultCnt/1
  Constant1/1 -> FaultDetected/1

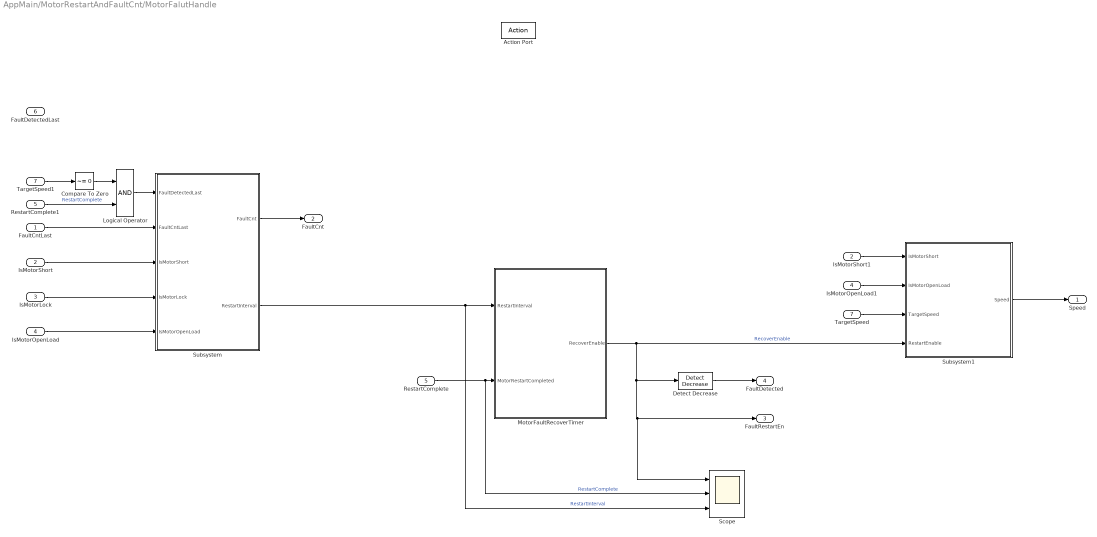
== system AppMain/MotorRestartAndFaultCnt/MotorFalutHandle ==
  FaultCntLast : Inport  OutDataTypeStr=Bus: MotorFaultCnt_t
  IsMotorShort : Inport  Port=2  OutDataTypeStr=boolean
  IsMotorLock : Inport  Port=3  OutDataTypeStr=boolean
  IsMotorOpenLoad : Inport  Port=4  OutDataTypeStr=boolean
  RestartComplete : Inport  Port=5  OutDataTypeStr=boolean
  FaultDetectedLast : Inport  Port=6  OutDataTypeStr=boolean
  TargetSpeed : Inport  Port=7  OutDataTypeStr=int16
  Action Port : ActionPort  InitializeStates=reset  ActionPortLabel=elseif(u2 ~= 0)
  Compare To Zero : simulink/Logic and Bit Operations/Compare To Zero  relop=~=  OutDataTypeStr=boolean
  Detect Decrease : simulink/Logic and Bit Operations/Detect Decrease  vinit=0.0  OutDataTypeStr=boolean
  IsMotorOpenLoad1 : InportShadow  Port=4  OutDataTypeStr=boolean
  IsMotorShort1 : InportShadow  Port=2  OutDataTypeStr=boolean
  Logical Operator : Logic  AllPortsSameDT=off  OutDataTypeStr=boolean
  MotorFaultRecoverTimer : Subsystem  TreatAsAtomicUnit=on
  RestartComplete1 : InportShadow  Port=5  OutDataTypeStr=boolean
  Scope : Scope  NumInputPorts=3
  Subsystem : Subsystem
  Subsystem1 : Subsystem
  TargetSpeed1 : InportShadow  Port=7  OutDataTypeStr=int16
  Speed : Outport  OutDataTypeStr=int16  VectorParamsAs1DForOutWhenUnconnected=off
  FaultCnt : Outport  Port=2  OutDataTypeStr=Bus: MotorFaultCnt_t  VectorParamsAs1DForOutWhenUnconnected=off
  FaultRestartEn : Outport  Port=3  OutDataTypeStr=boolean  VectorParamsAs1DForOutWhenUnconnected=off
  FaultDetected : Outport  Port=4  OutDataTypeStr=boolean  VectorParamsAs1DForOutWhenUnconnected=off
  wires:
  MotorFaultRecoverTimer/1(RecoverEnable) -> Scope/1, FaultRestartEn/1, Detect Decrease/1, Subsystem1/4(RestartEnable)  "RecoverEnable"
  Detect Decrease/1 -> FaultDetected/1
  FaultCntLast/1 -> Subsystem/2(FaultCntLast)
  IsMotorShort/1 -> Subsystem/3(IsMotorShort)
  IsMotorLock/1 -> Subsystem/4(IsMotorLock)
  IsMotorOpenLoad/1 -> Subsystem/5(IsMotorOpenLoad)
  Subsystem/1(FaultCnt) -> FaultCnt/1
  Subsystem/2(RestartInterval) -> Scope/3, MotorFaultRecoverTimer/1(RestartInterval)  "RestartInterval"
  RestartComplete/1 -> Scope/2, MotorFaultRecoverTimer/2(MotorRestartCompleted)  "RestartComplete"
  TargetSpeed/1 -> Subsystem1/3(TargetSpeed)
  Subsystem1/1(Speed) -> Speed/1
  Logical Operator/1 -> Subsystem/1(FaultDetectedLast)
  Compare To Zero/1 -> Logical Operator/1
  TargetSpeed1/1 -> Compare To Zero/1
  RestartComplete1/1 -> Logical Operator/2  "RestartComplete"
  IsMotorShort1/1 -> Subsystem1/1(IsMotorShort)
  IsMotorOpenLoad1/1 -> Subsystem1/2(IsMotorOpenLoad)

== system AppMain/MotorRestartAndFaultCnt/Normal ==
  TargetSpeed : Inport  OutDataTypeStr=int16
  Action Port : ActionPort  ActionPortLabel=else
  Bus Creator : BusCreator  Inputs=3  OutDataTypeStr=Bus: MotorFaultCnt_t  NonVirtualBus=on
      settings: InheritFromInputs=off
  Constant : Constant  Value=0  OutDataTypeStr=uint8
  Constant1 : Constant  OutDataTypeStr=boolean
  Constant2 : Constant  Value=0  OutDataTypeStr=boolean
  Constant3 : Constant  Value=0  OutDataTypeStr=uint8
  Constant4 : Constant  Value=0  OutDataTypeStr=uint8
  Speed : Outport  OutDataTypeStr=int16  VectorParamsAs1DForOutWhenUnconnected=off
  FaultRestartEn : Outport  Port=2  OutDataTypeStr=boolean  VectorParamsAs1DForOutWhenUnconnected=off
  FaultCnt : Outport  Port=3  OutDataTypeStr=Bus: MotorFaultCnt_t  VectorParamsAs1DForOutWhenUnconnected=off
  FaultDetected : Outport  Port=4  OutDataTypeStr=boolean  VectorParamsAs1DForOutWhenUnconnected=off
  wires:
  Constant2/1 -> FaultRestartEn/1
  Bus Creator/1 -> FaultCnt/1  "FaultCntRst"
  TargetSpeed/1 -> Speed/1
  Constant1/1 -> FaultDetected/1
  Constant3/1 -> Bus Creator/2  "Open"
  Constant/1 -> Bus Creator/1  "Short"
  Constant4/1 -> Bus Creator/3  "Lock"

== system AppMain/PwmInParamEval/PwmInshortDetect ==
  PwmInIdleTime : Inport  OutDataTypeStr=uint16
  PwmInPinState : Inport  Port=2  OutDataTypeStr=boolean
  Logical Operator : Logic  AllPortsSameDT=off  OutDataTypeStr=boolean
  Logical Operator1 : Logic  AllPortsSameDT=off  OutDataTypeStr=boolean
  Logical Operator2 : Logic  Operator=NOT  AllPortsSameDT=off  OutDataTypeStr=boolean
  PwmInBusTimeOutCntTHR : Constant  Value=CtrlConst.PwmIn.BusTimeOutCntTHR  OutDataTypeStr=uint16
  Relational Operator : RelationalOperator  OutDataTypeStr=boolean  RndMeth=Simplest
  shortGND : Outport  OutDataTypeStr=boolean  VectorParamsAs1DForOutWhenUnconnected=off
  shortBat : Outport  Port=2  VectorParamsAs1DForOutWhenUnconnected=off
  wires:
  PwmInPinState/1 -> Logical Operator/2, Logical Operator2/1
  PwmInBusTimeOutCntTHR/1 -> Relational Operator/2
  Logical Operator1/1 -> shortGND/1  "ShortGND"
  PwmInIdleTime/1 -> Relational Operator/1
  Relational Operator/1 -> Logical Operator1/1, Logical Operator/1
  Logical Operator/1 -> shortBat/1  "ShortBat"
  Logical Operator2/1 -> Logical Operator1/2

== system AppMain/PwmInTargetSpeedEval/NormalState ==
  PowerOnCntIn : Inport  OutDataTypeStr=uint16
  PwmInStatus : Inport  Port=2
  FilteredVoltage : Inport  Port=3  OutDataTypeStr=int16
  IsPwmDutyUpdated : Inport  Port=4  OutDataTypeStr=boolean
  Action Port : ActionPort  ActionPortLabel=else
  PwmInSpeedCtrl : Subsystem  TreatAsAtomicUnit=on
      settings: RTWFcnNameOpts=Use subsystem name
  PowerOnCntOut : Outport  VectorParamsAs1DForOutWhenUnconnected=off
  TargetSpeed : Outport  Port=2  VectorParamsAs1DForOutWhenUnconnected=off
  PwmInError : Outport  Port=3  OutDataTypeStr=boolean  VectorParamsAs1DForOutWhenUnconnected=off
  wires:
  PwmInSpeedCtrl/2(PwmInError) -> PwmInError/1
  PwmInSpeedCtrl/1(PwmInTargetSpeed) -> TargetSpeed/1  "PwmInCtrlSpeed"
  PwmInStatus/1 -> PwmInSpeedCtrl/1(PwmInStatus)
  PowerOnCntIn/1 -> PowerOnCntOut/1
  FilteredVoltage/1 -> PwmInSpeedCtrl/2(FilteredVoltage)
  IsPwmDutyUpdated/1 -> PwmInSpeedCtrl/3(IsPwmDutyUpdated)  "IsPwmDutyUpdated"

== system AppMain/PwmInTargetSpeedEval/PowerOnBlankState ==
  PowerOnCntIn : Inport  OutDataTypeStr=uint16
  Action Port : ActionPort  ActionPortLabel=if(u1 ~= 0)
  Add : Sum
  AddOne : Constant  OutDataTypeStr=uint16  SampleTime=-1
  InitErrSts : Constant  Value=0  OutDataTypeStr=boolean  SampleTime=-1
  InitSpeed : Constant  Value=0  OutDataTypeStr=int16  SampleTime=-1
  PowerOnCntOut : Outport  VectorParamsAs1DForOutWhenUnconnected=off
  TargetSpeed : Outport  Port=2  OutDataTypeStr=int16  VectorParamsAs1DForOutWhenUnconnected=off
  PwmInError : Outport  Port=3  OutDataTypeStr=boolean  VectorParamsAs1DForOutWhenUnconnected=off
  wires:
  InitSpeed/1 -> TargetSpeed/1  "InitSpeed"
  InitErrSts/1 -> PwmInError/1
  PowerOnCntIn/1 -> Add/2  "PowerOnCntLast"
  AddOne/1 -> Add/1
  Add/1 -> PowerOnCntOut/1  "PowerOnCnt"

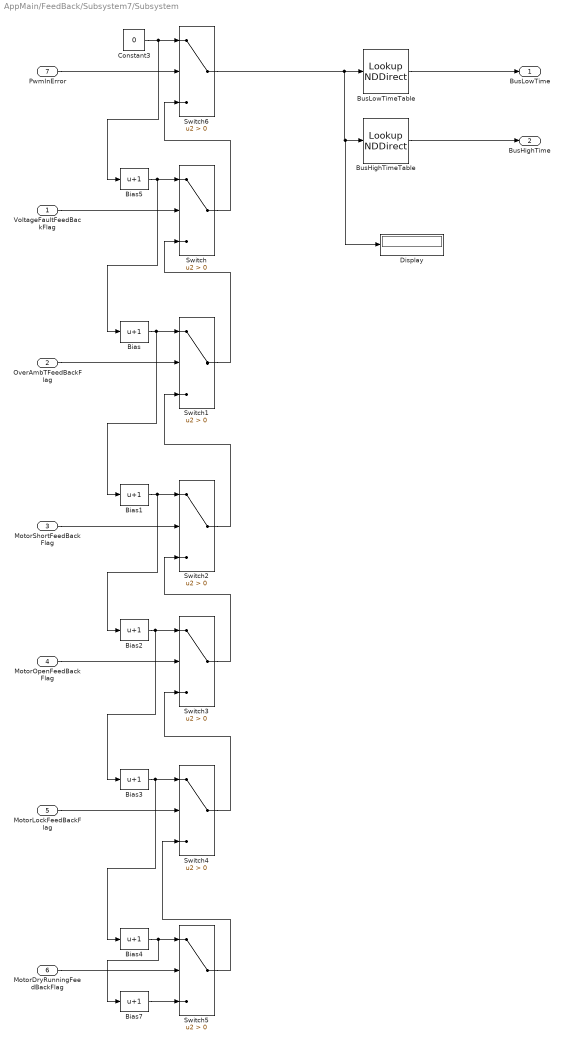
== system AppMain/FeedBack/Subsystem7/Subsystem ==
  VoltageFaultFeedBackFlag : Inport  OutDataTypeStr=boolean
  OverAmbTFeedBackFlag : Inport  Port=2  OutDataTypeStr=boolean
  MotorShortFeedBackFlag : Inport  Port=3  OutDataTypeStr=boolean
  MotorOpenFeedBackFlag : Inport  Port=4  OutDataTypeStr=boolean
  MotorLockFeedBackFlag : Inport  Port=5  OutDataTypeStr=boolean
  MotorDryRunningFeedBackFlag : Inport  Port=6  OutDataTypeStr=boolean
  PwmInError : Inport  Port=7  OutDataTypeStr=boolean
  Bias{,1..5,7} (7 alike) : Bias  Bias=1
  BusHighTimeTable : LookupNDDirect  NumberOfTableDimensions=1  Table=[CtrlConst.FeedBack.HighTime.PwmInError,CtrlConst.FeedBack.HighTime.Voltage,CtrlConst.FeedBack.HighTime.AmbT,CtrlConst.FeedBack.HighTime.MotorShort,CtrlConst.FeedBack.HighTime.MotorOpenLoad,CtrlConst.FeedBack.HighTime.MotorLock,CtrlConst.FeedBack.HighTime.MotorDryRunning,CtrlConst.FeedBack.HighTime.Normal]  TableDataTypeStr=uint16
  BusLowTimeTable : LookupNDDirect  NumberOfTableDimensions=1  Table=[CtrlConst.FeedBack.LowTime.PwmInError,CtrlConst.FeedBack.LowTime.Voltage,CtrlConst.FeedBack.LowTime.AmbT,CtrlConst.FeedBack.LowTime.MotorShort,CtrlConst.FeedBack.LowTime.MotorOpenLoad,CtrlConst.FeedBack.LowTime.MotorLock,CtrlConst.FeedBack.LowTime.MotorDryRunning,CtrlConst.FeedBack.LowTime.Normal]  TableDataTypeStr=uint16
  Constant3 : Constant  Value=0  OutDataTypeStr=uint16
  Display : Display
  Switch{,1..6} (7 alike) : Switch  Criteria=u2 > Threshold  OutDataTypeStr=uint16
  BusLowTime : Outport  VectorParamsAs1DForOutWhenUnconnected=off
  BusHighTime : Outport  Port=2  VectorParamsAs1DForOutWhenUnconnected=off
  wires:
  Switch6/1 -> BusHighTimeTable/1, Display/1, BusLowTimeTable/1
  Switch1/1 -> Switch/3
  Bias4/1 -> Bias7/1, Switch5/1
  Switch5/1 -> Switch4/3
  Switch3/1 -> Switch2/3
  Switch4/1 -> Switch3/3
  Bias2/1 -> Bias3/1, Switch3/1
  Bias3/1 -> Bias4/1, Switch4/1
  Bias/1 -> Bias1/1, Switch1/1
  OverAmbTFeedBackFlag/1 -> Switch1/2
  Switch2/1 -> Switch1/3
  Bias1/1 -> Bias2/1, Switch2/1
  VoltageFaultFeedBackFlag/1 -> Switch/2
  MotorOpenFeedBackFlag/1 -> Switch3/2
  MotorDryRunningFeedBackFlag/1 -> Switch5/2
  MotorLockFeedBackFlag/1 -> Switch4/2
  MotorShortFeedBackFlag/1 -> Switch2/2
  BusHighTimeTable/1 -> BusHighTime/1
  Bias7/1 -> Switch5/3
  BusLowTimeTable/1 -> BusLowTime/1
  PwmInError/1 -> Switch6/2
  Bias5/1 -> Bias/1, Switch/1
  Constant3/1 -> Bias5/1, Switch6/1
  Switch/1 -> Switch6/3

== system AppMain/FeedBack/Subsystem7/Subsystem1 ==
  VoltageStatus : Inport
  Compare To Zero : simulink/Logic and Bit Operations/Compare To Zero  relop=~=  OutDataTypeStr=boolean
  Constant1 : Constant  Value=CtrlConst.FeedBack.EndDelay.Voltage  OutDataTypeStr=uint16
  Constant2 : Constant  Value=CtrlConst.FeedBack.StartDelay.Voltage  OutDataTypeStr=uint16
  Display : Display
  Display1 : Display
  FeedBackDelay4 : lib1/FeedBackDelay  SystemSampleTime=-1  VariantActivationTime=update diagram  Latency=0  AutoFrameSizeCalculation=off
      settings: SourceProductName=lib1
  VoltageFaultFeedBackFlag : Outport  VectorParamsAs1DForOutWhenUnconnected=off
  wires:
  FeedBackDelay4/1 -> VoltageFaultFeedBackFlag/1  "VoltageFaultFeedBackFlag"
  Constant1/1 -> Display1/1, FeedBackDelay4/3
  Constant2/1 -> Display/1, FeedBackDelay4/1
  Compare To Zero/1 -> FeedBackDelay4/2
  VoltageStatus/1 -> Compare To Zero/1

== system AppMain/FeedBack/Subsystem7/Subsystem2 ==
  AmbTStatus : Inport
  Compare To Zero1 : simulink/Logic and Bit Operations/Compare To Zero  relop=>  OutDataTypeStr=boolean
  Constant4 : Constant  Value=CtrlConst.FeedBack.StartDelay.AmbT  OutDataTypeStr=uint16
  Constant5 : Constant  Value=CtrlConst.FeedBack.EndDelay.AmbT  OutDataTypeStr=uint16
  FeedBackDelay5 : lib1/FeedBackDelay  SystemSampleTime=-1  VariantActivationTime=update diagram  Latency=0  AutoFrameSizeCalculation=off
      settings: SourceProductName=lib1
  OverAmbTFeedBackFlag : Outport  VectorParamsAs1DForOutWhenUnconnected=off
  wires:
  Compare To Zero1/1 -> FeedBackDelay5/2
  AmbTStatus/1 -> Compare To Zero1/1
  Constant5/1 -> FeedBackDelay5/3
  Constant4/1 -> FeedBackDelay5/1
  FeedBackDelay5/1 -> OverAmbTFeedBackFlag/1  "OverAmbTFeedBackFlag"

== system AppMain/FeedBack/Subsystem7/Subsystem3 ==
  FaultFlag : Inport  OutDataTypeStr=boolean
  FaultCnt : Inport  Port=2  OutDataTypeStr=uint8
  MotorRunEn : Inport  Port=3
  Compare To Constant : simulink/Logic and Bit Operations/Compare To Constant  relop=>=  const=20  OutDataTypeStr=boolean
  FeedBackEnLast : Memory  InheritSampleTime=on
  Logical Operator : Logic  Inputs=3  AllPortsSameDT=off  OutDataTypeStr=boolean
  Logical Operator1 : Logic  AllPortsSameDT=off  OutDataTypeStr=boolean
  Logical Operator3 : Logic  Operator=OR  AllPortsSameDT=off  OutDataTypeStr=boolean
  FeedBackEn : Outport  VectorParamsAs1DForOutWhenUnconnected=off
  wires:
  Compare To Constant/1 -> Logical Operator3/2
  FaultFlag/1 -> Logical Operator/1, Logical Operator1/1
  Logical Operator3/1 -> FeedBackEnLast/1, Logical Operator/2
  Logical Operator/1 -> FeedBackEn/1
  MotorRunEn/1 -> Logical Operator/3
  FaultCnt/1 -> Compare To Constant/1
  FeedBackEnLast/1 -> Logical Operator1/2
  Logical Operator1/1 -> Logical Operator3/1

== system AppMain/FeedBack/Subsystem7/Subsystem4 ==
  FaultFlag : Inport  OutDataTypeStr=boolean
  FaultCnt : Inport  Port=2  OutDataTypeStr=uint8
  MotorRunEn : Inport  Port=3
  Compare To Constant : simulink/Logic and Bit Operations/Compare To Constant  relop=>=  const=20  OutDataTypeStr=boolean
  FeedBackEnLast : Memory  InheritSampleTime=on
  Logical Operator : Logic  Inputs=3  AllPortsSameDT=off  OutDataTypeStr=boolean
  Logical Operator1 : Logic  AllPortsSameDT=off  OutDataTypeStr=boolean
  Logical Operator3 : Logic  Operator=OR  AllPortsSameDT=off  OutDataTypeStr=boolean
  FeedBackEn : Outport  VectorParamsAs1DForOutWhenUnconnected=off
  wires:
  Compare To Constant/1 -> Logical Operator3/2
  FaultFlag/1 -> Logical Operator/1, Logical Operator1/1
  Logical Operator3/1 -> FeedBackEnLast/1, Logical Operator/2
  Logical Operator/1 -> FeedBackEn/1
  MotorRunEn/1 -> Logical Operator/3
  FaultCnt/1 -> Compare To Constant/1
  FeedBackEnLast/1 -> Logical Operator1/2
  Logical Operator1/1 -> Logical Operator3/1

== system AppMain/FeedBack/Subsystem7/Subsystem5 ==
  FaultFlag : Inport  OutDataTypeStr=boolean
  FaultCnt : Inport  Port=2  OutDataTypeStr=uint8
  MotorRunEn : Inport  Port=3
  Compare To Constant : simulink/Logic and Bit Operations/Compare To Constant  relop=>=  const=20  OutDataTypeStr=boolean
  FeedBackEnLast : Memory  InheritSampleTime=on
  Logical Operator : Logic  Inputs=3  AllPortsSameDT=off  OutDataTypeStr=boolean
  Logical Operator1 : Logic  AllPortsSameDT=off  OutDataTypeStr=boolean
  Logical Operator3 : Logic  Operator=OR  AllPortsSameDT=off  OutDataTypeStr=boolean
  FeedBackEn : Outport  VectorParamsAs1DForOutWhenUnconnected=off
  wires:
  Compare To Constant/1 -> Logical Operator3/2
  FaultFlag/1 -> Logical Operator/1, Logical Operator1/1
  Logical Operator3/1 -> FeedBackEnLast/1, Logical Operator/2
  Logical Operator/1 -> FeedBackEn/1
  MotorRunEn/1 -> Logical Operator/3
  FaultCnt/1 -> Compare To Constant/1
  FeedBackEnLast/1 -> Logical Operator1/2
  Logical Operator1/1 -> Logical Operator3/1

== system AppMain/MotorRestartAndFaultCnt/MotorFalutHandle/MotorFaultRecoverTimer ==
  RestartInterval : Inport  OutDataTypeStr=uint16
  MotorRestartCompleted : Inport  Port=2
  MotorRestartFSM : Stateflow chart  TreatAsAtomicUnit=on
  RecoverEnable : Outport  VectorParamsAs1DForOutWhenUnconnected=off
  wires:
  MotorRestartCompleted/1 -> MotorRestartFSM/2(MotorRestartCompleted)
  MotorRestartFSM/1(RecoverEn) -> RecoverEnable/1
  RestartInterval/1 -> MotorRestartFSM/1(TimeTHR)

== system AppMain/MotorRestartAndFaultCnt/MotorFalutHandle/Subsystem ==
  FaultDetectedLast : Inport  OutDataTypeStr=boolean
  FaultCntLast : Inport  Port=2  OutDataTypeStr=Bus: MotorFaultCnt_t
  IsMotorShort : Inport  Port=3  OutDataTypeStr=boolean
  IsMotorLock : Inport  Port=4  OutDataTypeStr=boolean
  IsMotorOpenLoad : Inport  Port=5  OutDataTypeStr=boolean
  FaultCntLast1 : InportShadow  Port=2  OutDataTypeStr=Bus: MotorFaultCnt_t
  If : If  IfExpression=u1 ~= 0
  If Action Subsystem : Subsystem  TreatAsAtomicUnit=on
  If Action Subsystem1 : Subsystem  TreatAsAtomicUnit=on
  Merge : Merge
  Merge1 : Merge
  RestartIntervalLast : Memory  InheritSampleTime=on
  FaultCnt : Outport  OutDataTypeStr=Bus: MotorFaultCnt_t  VectorParamsAs1DForOutWhenUnconnected=off
  RestartInterval : Outport  Port=2  OutDataTypeStr=uint16  VectorParamsAs1DForOutWhenUnconnected=off
  wires:
  RestartIntervalLast/1 -> If Action Subsystem1/2(RestartIntervalLast)  "RestartIntervalLast"
  If Action Subsystem1/2(RestartInterval) -> Merge1/2
  If Action Subsystem1/1(FaultCnt) -> Merge/2
  If/1 -> If Action Subsystem/Action
  If/2 -> If Action Subsystem1/Action
  Merge1/1 -> RestartIntervalLast/1, RestartInterval/1  "RestartInterval"
  FaultCntLast/1 -> If Action Subsystem/1(FalutCntLast)
  If Action Subsystem/1(FaultCnt) -> Merge/1
  Merge/1 -> FaultCnt/1  "FaultCnt"
  If Action Subsystem/2(RestartInterval) -> Merge1/1
  FaultDetectedLast/1 -> If/1
  IsMotorShort/1 -> If Action Subsystem/2(IsMotorShort)
  IsMotorLock/1 -> If Action Subsystem/3(IsMotorLock)
  IsMotorOpenLoad/1 -> If Action Subsystem/4(IsMotorOpenLoad)
  FaultCntLast1/1 -> If Action Subsystem1/1(FaultCntLast)

== system AppMain/MotorRestartAndFaultCnt/MotorFalutHandle/Subsystem1 ==
  IsMotorShort : Inport  OutDataTypeStr=boolean
  IsMotorOpenLoad : Inport  Port=2  OutDataTypeStr=boolean
  TargetSpeed : Inport  Port=3  OutDataTypeStr=int16
  RestartEnable : Inport  Port=4  OutDataTypeStr=boolean
  If : If  IfExpression=u1 ~= 0
  If Action Subsystem : Subsystem  TreatAsAtomicUnit=on
  If Action Subsystem1 : Subsystem  TreatAsAtomicUnit=on
  Logical Operator : Logic  Operator=OR  AllPortsSameDT=off  OutDataTypeStr=boolean
  Merge : Merge
  Scope : Scope
  Speed : Outport  OutDataTypeStr=int16  VectorParamsAs1DForOutWhenUnconnected=off
  wires:
  IsMotorShort/1 -> Logical Operator/1
  IsMotorOpenLoad/1 -> Logical Operator/2
  Logical Operator/1 -> If/1
  TargetSpeed/1 -> If Action Subsystem1/1(SpeedIn), If Action Subsystem/1(SpeedIn)
  RestartEnable/1 -> If Action Subsystem1/2(RestartEnable)
  If/1 -> If Action Subsystem/Action
  If/2 -> If Action Subsystem1/Action
  If Action Subsystem1/1(SpeedOut) -> Merge/2
  If Action Subsystem/1(SpeedOut) -> Merge/1
  Merge/1 -> Speed/1, Scope/1
